simulink model "mppt_2"  (R2023b)
settings: Solver=VariableStepAuto  StartTime=0.0  StopTime=10.0  RelTol=1e-3
libraries: spsSeriesRLCBranchLib x4, spsCurrentMeasurementLib x1, spsDiodeLib x1, spsGroundLib x1, spsIGBTDiodeLib x1, spsPVArrayLib x1, spsSawtoothGeneratorLib x1, spsVoltageMeasurementLib x1, sps_lib x1
settings Model: Creator=user  LastModifiedBy=user

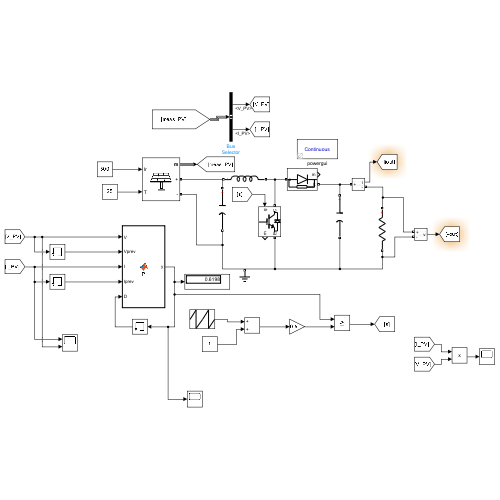
[thumbnail: Simulink's stored preview of the top-level diagram]
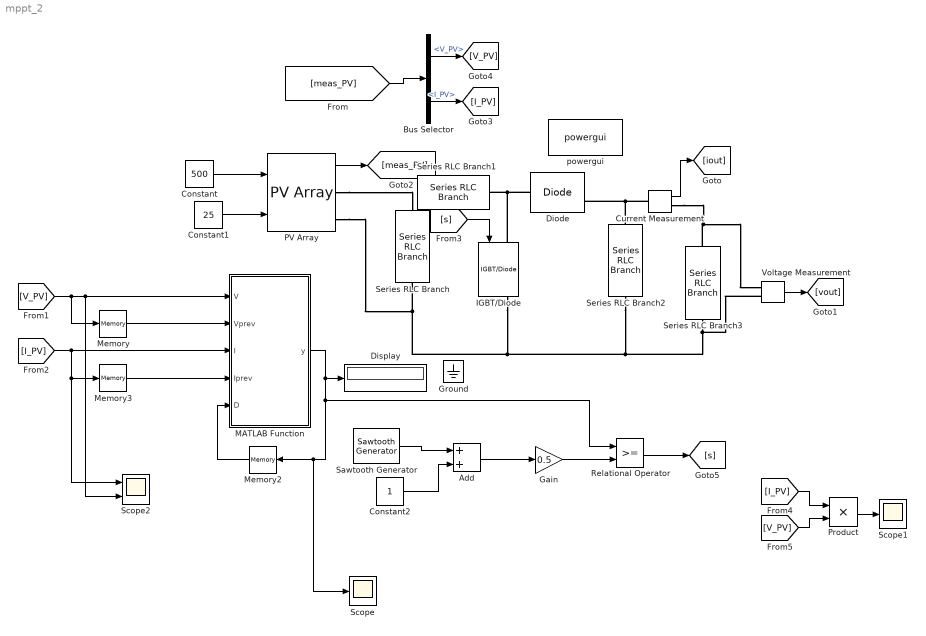
== system mppt_2 ==
  Add : Sum
  Bus Selector : BusSelector  OutputSignals=V_PV,I_PV
  Constant : Constant  Value=500
  Constant1 : Constant  Value=25
  Constant2 : Constant
  Current Measurement : spsCurrentMeasurementLib/Current Measurement  PhasorSimulation=off  OutputType=Complex  PSBequivalent=0
  Diode : spsDiodeLib/Diode  Ron=0.001  Lon=0  Vf=0.8  IC=0  UseSnubber=0  Rs=500  Cs=250e-9  Measurements=on
  Display : Display
  Gain : Gain  Gain=0.5
  Ground : spsGroundLib/Ground  LConnTagsString=a
  IGBT/Diode : spsIGBTDiodeLib/IGBT//Diode  Ron=1e-3  Rs=1e5  Cs=inf  Measurements=on
  MATLAB Function : MATLAB Function  TreatAsAtomicUnit=on
  Memory : Memory
  Memory2 : Memory
  Memory3 : Memory
  PV Array : spsPVArrayLib/PV Array  Npar=5  Nser=33  PlotType=array @ 25 deg.C & specified irradiances  S_vec="[ 1000  500  100 ]"  Temp_C_vec="[ 45 25  ]"  ModuleName=Trina Solar TSM-250PA05.08  PlotWhenSelected=off  Pm=249.86  Ncell=60  Voc=37.6  Isc=8.55  Vm=31  Im=8.06  beta_Voc_pc=-0.35  alpha_Isc_pc=0.06  beta_Voc=-0.1316  alpha_Isc=0.00513  IL=8.5795  I0=2.0381e-10  nI=0.99766  Rsh=301.8149  Rs=0.247  RobustModel=off  RobustCellTemperature=313.3991  BAL=on  Tc=1e-6  Tfilter=5e-5
  Product : Product
  Relational Operator : RelationalOperator  OutDataTypeStr=boolean  RndMeth=Simplest  InputSameDT=off
  Sawtooth Generator : spsSawtoothGeneratorLib/Sawtooth Generator  Freq=1e3  Phase=180  Ts=0
  Scope : Scope
  Scope1 : Scope
  Scope2 : Scope  NumInputPorts=2
  Series RLC Branch : spsSeriesRLCBranchLib/Series RLC Branch  LConnTagsString=__new0  RConnTagsString=__new0  BranchType=C  Resistance=1  Inductance=1e-3  SetiL0=off  InitialCurrent=0  Capacitance=1e-6  Setx0=off  InitialVoltage=0  Measurements=None
  Series RLC Branch1 : spsSeriesRLCBranchLib/Series RLC Branch  LConnTagsString=__new0  RConnTagsString=__new0  BranchType=L  Resistance=1  Inductance=80e-3  SetiL0=off  InitialCurrent=0  Capacitance=1e-6  Setx0=off  InitialVoltage=0  Measurements=None
  Series RLC Branch2 : spsSeriesRLCBranchLib/Series RLC Branch  LConnTagsString=__new0  RConnTagsString=__new0  BranchType=C  Resistance=1  Inductance=1e-3  SetiL0=off  InitialCurrent=0  Capacitance=5000e-6  Setx0=off  InitialVoltage=0  Measurements=None
  Series RLC Branch3 : spsSeriesRLCBranchLib/Series RLC Branch  LConnTagsString=__new0  RConnTagsString=__new0  BranchType=R  Resistance=5  Inductance=80e-3  SetiL0=off  InitialCurrent=0  Capacitance=1e-6  Setx0=off  InitialVoltage=0  Measurements=None
  Voltage Measurement : spsVoltageMeasurementLib/Voltage Measurement  PhasorSimulation=off  OutputType=Complex  PSBequivalent=0
  powergui : sps_lib/powergui  Priority=1  SimulationMode=Continuous  SampleTime=50e-6  frequency=60  Iterations=50  frequencyindice=0  Pbase=100e6  ErrMax=1e-4  UnitsV=kV  UnitsW=MW  buscounter=0  FunctionMessages=off  echomessages=off  EnableUseOfTLC=off  CurrentSourceSwitches=off  DisableSnubberDevices=off  DisableRonSwitches=off  DisableVfSwitches=off  DisplayEquations=off  AutomaticDiscreteSolvers=off  SolverType=Tustin/Backward Euler (TBE)  Interpol=off  ExternalGateDelay=off  methode=off  Ts=100  x0status=blocks  SPID=on  SwTol=0  HookPort=off  NonlinearTolerance=1e-4  nMaxIteration=100  ContinueOnMaxIteration=off  RestoreLinks=warning  ResistiveCurrentMeasurement=off  Frange=[0:2:500]  Ylog=off  Xlog=on  ShowGrid=off  save=off  variable=ZData  structure=0  ZoomFFT=off  StartTime=0.0  cycles=1  DisplayStyle=1  fundamental=60  FreqAxis=off  MaxFrequency=1000  frequencyindicesteady=1  RmsSteady=1  display=off
  wires:
  Constant/1 -> PV Array/1
  Constant1/1 -> PV Array/2
  Current Measurement/1 -> [iout]
  Voltage Measurement/1 -> [vout]
  Sawtooth Generator/1 -> Add/1
  Constant2/1 -> Add/2
  Add/1 -> Gain/1
  Gain/1 -> Relational Operator/2
  PV Array/1 -> [meas_PV]
  [meas_PV] -> Bus Selector/1
  Bus Selector/1 -> [V_PV]  "<V_PV>"
  Bus Selector/2 -> [I_PV]  "<I_PV>"
  MATLAB Function/1(y) -> Display/1, Scope/1, Memory2/1, Relational Operator/1
  Memory2/1 -> MATLAB Function/5(D)
  [V_PV] -> Scope2/2, MATLAB Function/1(V), Memory/1
  Memory/1 -> MATLAB Function/2(Vprev)
  [I_PV] -> Scope2/1, Memory3/1, MATLAB Function/3(I)
  Memory3/1 -> MATLAB Function/4(Iprev)
  Relational Operator/1 -> [s]
  [s] -> IGBT/Diode/1
  Product/1 -> Scope1/1
  [V_PV] -> Product/2
  [I_PV] -> Product/1
  connections:
  PV Array/RConn1 -- Series RLC Branch/LConn1
  PV Array/RConn2 -- Voltage Measurement/LConn2 -- Series RLC Branch3/RConn1 -- Series RLC Branch2/RConn1 -- IGBT/Diode/RConn1 -- Series RLC Branch/RConn1
  IGBT/Diode/LConn1 -- Series RLC Branch1/RConn1 -- Diode/LConn1
  Series RLC Branch3/LConn1 -- Current Measurement/RConn1 -- Voltage Measurement/LConn1
  Series RLC Branch2/LConn1 -- Diode/RConn1 -- Current Measurement/LConn1

== matlab function mppt_2/MATLAB Function ==
  data: V input; y output; Vprev input; I input; Iprev input; D input
function y  = P(V, Vprev, I, Iprev, D)

if D == 0
    D = 0.5;
end
% step is anything you want..?
delta_D = 0.0001;
% input D is D_prev.. 

dI = I - Iprev;
dV = V - Vprev;

if dV == 0
    if dI == 0
        y = D;
    else
        if dI > 0
            y = D - delta_D;  
        else
            y = D + delta_D;
        end
    end
else
    if (I + (dI/dV)*V) == 0
        y = D;
    else
        if (I + (dI/dV)*V) > 0
            y = D - delta_D;
        else
            y = D + delta_D;
        end
    end
end
end
